simulink model "e1"  (R2014b)
settings: Solver=ode45  StartTime=0.0  StopTime=10.0  RelTol=1e-3
settings Model: Creator=Administrator  LastModifiedBy=Administrator

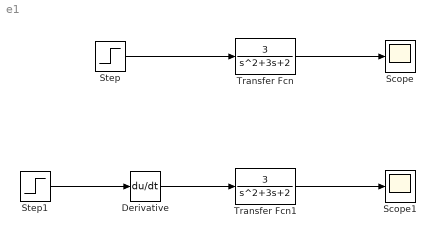
== system e1 ==
  Derivative : Derivative
  Scope : Scope
  Scope1 : Scope
  Step : Step  SampleTime=0
  Step1 : Step  SampleTime=0
  Transfer Fcn : TransferFcn  Numerator=[3]  Denominator=[1 3 2]
  Transfer Fcn1 : TransferFcn  Numerator=[3]  Denominator=[1 3 2]
  wires:
  Transfer Fcn/1 -> Scope/1
  Transfer Fcn1/1 -> Scope1/1
  Step1/1 -> Derivative/1
  Derivative/1 -> Transfer Fcn1/1
  Step/1 -> Transfer Fcn/1
